simulink model "untitled"  (R2015a)
settings: Solver=ode45  StartTime=0.0  StopTime=100  RelTol=1e-3
settings Model: Creator=ry0  LastModifiedBy=ry0

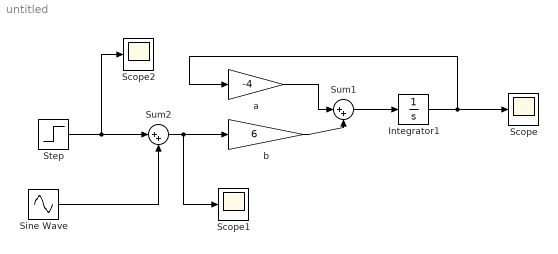
== system untitled ==
  Integrator1 : Integrator  InitialCondition=2
  Scope : Scope
  Scope1 : Scope
  Scope2 : Scope
      settings: SaveName=ScopeData2
  Sine Wave : Sin  Phase=pi/2  SampleTime=0
  Step : Step  Time=0  SampleTime=0
  Sum1 : Sum  Inputs=|++
  Sum2 : Sum  Inputs=|++
  a : Gain  Gain=-4
  b : Gain  Gain=6
  wires:
  Sum1/1 -> Integrator1/1
  Integrator1/1 -> Scope/1, a/1
  a/1 -> Sum1/1
  b/1 -> Sum1/2
  Sum2/1 -> Scope1/1, b/1
  Step/1 -> Scope2/1, Sum2/1
  Sine Wave/1 -> Sum2/2
